simulink model "TestModel_2024a"  (R2024a)
settings: Solver=FixedStepAuto  StartTime=0.0  StopTime=4  FixedStep=1e-6  RelTol=1e-3
values from neighbouring files (symbols this model uses):
  pmsm = mcb.getPMSMParameters('Teknic2310P')    [mcb_pmsm_foc_sensorless_f28379d_datascript.m]
  Ts = T_pwm    (= 5e-05)    [mcb_pmsm_foc_sensorless_f28379d_datascript.m]
  Ts_motor = T_pwm/2    (= 2.5e-05)    [mcb_pmsm_foc_sensorless_f28379d_datascript.m]
undefined symbols (not defined in the file or in its folder): DiscIntNeverNeededParam
libraries: mcbcontrolslib x3, spsCurrentMeasurementLib x1, autolibim x1, spsPWMGenerator2LevelLib x1, eePwmGeneratorTwoLevel x1, spsThreePhaseVIMeasurementLib x1, spsTwoLevelConverterLib x1, spsDCVoltageSourceLib x1, spsVoltageMeasurementLib x1, spspowerguiLib x1
settings Model: Creator=ckb527612  LastModifiedBy=ckb527612
settings ConfigComp: CovBoundaryAbsTol=1.0e-5

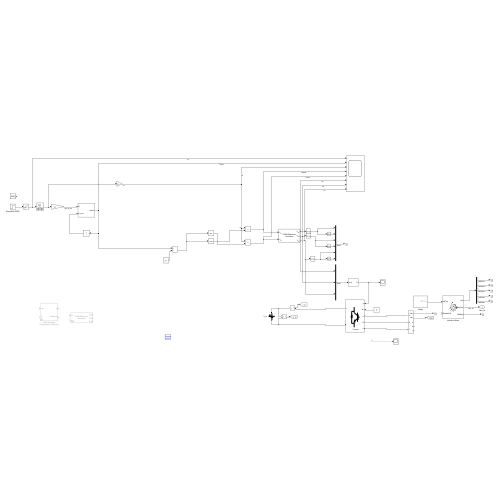
[thumbnail: Simulink's stored preview of the top-level diagram]
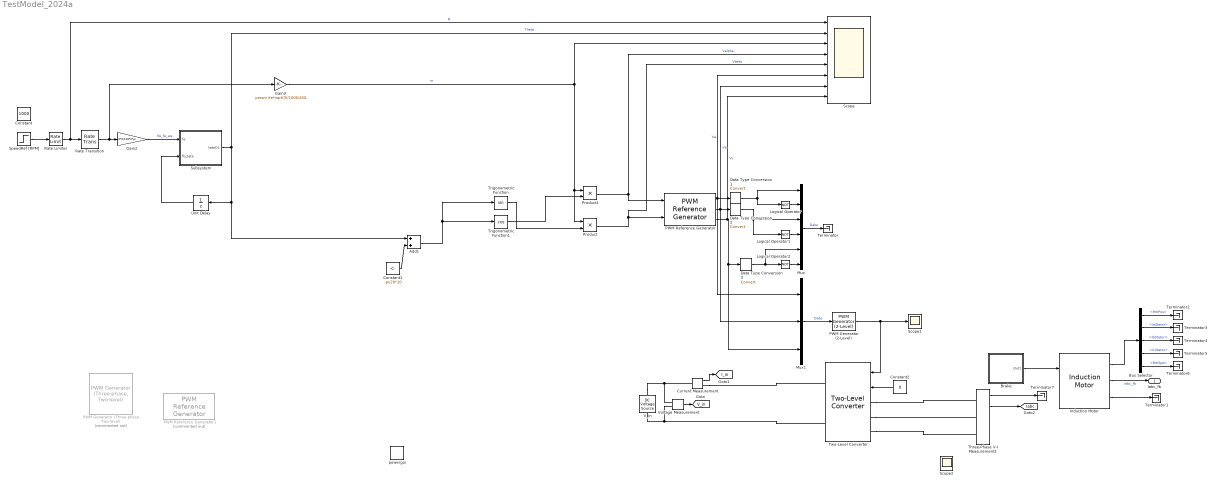
== system TestModel_2024a ==
  Add1 : Sum
  Brake : Subsystem
      mask Display: image('brake-system-types-and-hydraulic-brake-parts-and-functions-6.png');
  Bus Selector : BusSelector  OutputSignals=MtrPos,IaStator,IbStator,IcStator,MtrSpd
  Constant : Constant  Value=1000
  Constant1 : Constant  Value=-pi/20*10
  Constant2 : Constant  Value=0
  Current Measurement : spsCurrentMeasurementLib/Current Measurement  PhasorSimulation=off  OutputType=Complex  PSBequivalent=0
  Data Type Conversion1 : DataTypeConversion  SaturateOnIntegerOverflow=off  RndMeth=Floor
  Data Type Conversion2 : DataTypeConversion  SaturateOnIntegerOverflow=off  RndMeth=Floor
  Data Type Conversion3 : DataTypeConversion  SaturateOnIntegerOverflow=off  RndMeth=Floor
  Gain2 : Gain  Gain=2*2/120*2*pi
  Gain3 : Gain  Gain=pmsm.Ke*sqrt(3)/1000/450
  Induction Motor : autolibim/Induction Motor  sim_type=Discrete  Ts=0.001  port_config=Torque  P=2  Zs=[0.85 0.0139]  Zr="[0.55  0.0121]"  Lm=0.048  mechanical=[0.055 0.0078 0.5]  theta_init=0  omega_init=0  RefBlkName='autolibim/Induction Motor'  aMode=5
      settings: LibrarySourceBlock=mcblib/Electrical Systems/Motors/Induction Motor
  Logical Operator : Logic  Operator=NOT  AllPortsSameDT=off  OutDataTypeStr=boolean
  Logical Operator1 : Logic  Operator=NOT  AllPortsSameDT=off  OutDataTypeStr=boolean
  Logical Operator2 : Logic  Operator=NOT  AllPortsSameDT=off  OutDataTypeStr=boolean
  Mux : Mux  Inputs=6
  Mux1 : Mux  Inputs=3
  PWM Generator (2-Level) : spsPWMGenerator2LevelLib/PWM Generator (2-Level)  ModulatorType=Three-phase bridge (6 pulses)  ModulatorMode=Unsynchronized  Fc=10000  Pc=90  nF=27  MinMax="[ -1  1 ]"  SamplingTechnique=Natural  ModulatingSignals=off  m=0.8  Freq=60  Phase=0  Ts=1e-6  ShowCarrierOutport=off
  "PWM Generator (Three-phase, Two-level)" : eePwmGeneratorTwoLevel/PWM Generator (Three-phase, Two-level)  Commented=on  PWMMode=Continuous PWM (CPWM)  CPWMMode=SVM: space vector modulation  DPWMMode=60 DPWM: 60 degree discontinuous PWM  fsw=10e3  Ts=1e-6
      settings: LibrarySourceBlock=|
      | ee_sl_lib/Pulse Width
      | Modulation/PWM Generator
      | (Three-phase, Two-level)
  PWM Reference Generator : mcbcontrolslib/PWM Reference Generator  inSignal=Valphabeta  modType=SVM: space vector modulation
      settings: LibrarySourceBlock=mcblib/Controls/Math Transforms/PWM Reference Generator
  PWM Reference Generator1 : mcbcontrolslib/PWM Reference Generator  Commented=on  inSignal=Valphabeta  modType=SVM: space vector modulation
      settings: LibrarySourceBlock=mcblib/Controls/Math Transforms/PWM Reference Generator
  Product : Product
  Product1 : Product
  Rate Limiter : RateLimiter  RisingSlewLimit=1000  SampleTimeMode=inherited
  Rate Transition : RateTransition  OutPortSampleTime=5e-5
  Scope : Scope  NumInputPorts=8
  Scope1 : Scope
  Scope2 : Scope
  SpeedRef [RPM] : Step  Time=2  Before=500  After=1000  OutDataTypeStr=single  SampleTime=Ts
  Subsystem : Subsystem
  Terminator{,1..7} (8 alike) : Terminator
  Three-Phase V-I Measurement2 : spsThreePhaseVIMeasurementLib/Three-Phase V-I Measurement  VoltageMeasurement=phase-to-phase  SetLabelV=off  LabelV=Vabc  Vpu=off  VpuLL=off  CurrentMeasurement=yes  SetLabelI=off  LabelI=Iabc  Ipu=off  Pbase=100e6  Vbase=500e3  OutputType=Complex  PhasorSimulation=off  PSBequivalent=0
  Trigonometric Function : Trigonometry
  Trigonometric Function1 : Trigonometry  Operator=cos
  Two-Level Converter : spsTwoLevelConverterLib/Two-Level Converter  ModelType=Switching devices  Ron=1e-3  Rs=1e6  Cs=inf  Vforward=[0,0]  Ron_Diode=1e-3  Rs_Diode=1e6  Cs_Diode=inf  Vf_Diode=1e-3  Rs_CurrentSource=inf  Ron_ACsource=1e-3
      settings: LibrarySourceBlock=sps_lib/Power Electronics/Two-Level Converter
  Unit Delay : UnitDelay  SampleTime=-1  HasFrameUpgradeWarning=on
  "V_in " : spsDCVoltageSourceLib/DC Voltage Source  Amplitude=650  Measurements=None
  Voltage Measurement : spsVoltageMeasurementLib/Voltage Measurement  PhasorSimulation=off  OutputType=Complex  PSBequivalent=0
  powergui : spspowerguiLib/powergui  Priority=1  SimulationMode=Discrete  SampleTime=1e-6  frequency=60  Iterations=50  frequencyindice=0  Pbase=100e6  ErrMax=1e-4  UnitsV=kV  UnitsW=MW  buscounter=0  FunctionMessages=off  echomessages=off  EnableUseOfTLC=off  CurrentSourceSwitches=off  DisableSnubberDevices=off  DisableRonSwitches=off  DisableVfSwitches=off  DisplayEquations=off  AutomaticDiscreteSolvers=off  SolverType=Tustin/Backward Euler (TBE)  Interpol=off  ExternalGateDelay=off  methode=off  Ts=100  x0status=blocks  SPID=on  SwTol=0  HookPort=off  NonlinearTolerance=1e-4  nMaxIteration=100  ContinueOnMaxIteration=off  RestoreLinks=warning  ResistiveCurrentMeasurement=off  Frange=[0:2:500]  Ylog=off  Xlog=on  ShowGrid=off  save=off  variable=ZData  structure=0  ZoomFFT=off  StartTime=0.0  cycles=1  DisplayStyle=1  fundamental=60  FreqAxis=off  MaxFrequency=1000  frequencyindicesteady=1  RmsSteady=1  display=off
  Iabc_fb : Outport
  tag scope: I_in=global, Iabc=global, V_in=global
  wires:
  Unit Delay/1 -> Subsystem/2(fb_teta)
  Gain2/1 -> Subsystem/1(fe)  "Ns_fe_we"
  Rate Limiter/1 -> Scope/1, Rate Transition/1  "N"
  SpeedRef [RPM]/1 -> Rate Limiter/1
  Trigonometric Function1/1 -> Product1/2
  Data Type Conversion1/1 -> Logical Operator/1, Mux/1
  PWM Reference Generator/1 -> Mux1/1, Scope/6, Data Type Conversion1/1  "Va"
  Logical Operator1/1 -> Mux/4
  Data Type Conversion2/1 -> Logical Operator1/1, Mux/3
  Logical Operator2/1 -> Mux/6
  Product1/1 -> Scope/4, PWM Reference Generator/1  "Valpha"
  PWM Reference Generator/3 -> Scope/8, Mux1/3, Data Type Conversion3/1  "Vc"
  Trigonometric Function/1 -> Product/2
  PWM Reference Generator/2 -> Mux1/2, Scope/7, Data Type Conversion2/1  "Vb"
  Add1/1 -> Trigonometric Function1/1, Trigonometric Function/1
  Subsystem/1(tetaOL) -> Add1/1, Unit Delay/1, Scope/2  "Theta"
  Logical Operator/1 -> Mux/2
  Mux/1 -> Terminator/1  "Dabc"
  Product/1 -> Scope/5, PWM Reference Generator/2  "Vbeta"
  Data Type Conversion3/1 -> Mux/5, Logical Operator2/1
  Constant1/1 -> Add1/2
  Gain3/1 -> Product/1, Product1/1, Scope/3  "m"
  Rate Transition/1 -> Gain3/1, Gain2/1
  Mux1/1 -> PWM Generator (2-Level)/1  "Dabc"
  PWM Generator (2-Level)/1 -> Two-Level Converter/1, Scope1/1
  Constant2/1 -> Two-Level Converter/2
  Voltage Measurement/1 -> [V_in]
  Current Measurement/1 -> [I_in]
  Induction Motor/2 -> Iabc_fb/1  "Iabc_fb"
  Induction Motor/1 -> Bus Selector/1
  Three-Phase V-I Measurement2/1 -> Terminator7/1
  Three-Phase V-I Measurement2/2 -> [Iabc]
  Induction Motor/3 -> Terminator1/1
  Brake/1(Out1) -> Induction Motor/1
  Bus Selector/1 -> Terminator2/1  "<MtrPos>"
  Bus Selector/2 -> Terminator3/1  "<IaStator>"
  Bus Selector/3 -> Terminator4/1  "<IbStator>"
  Bus Selector/4 -> Terminator5/1  "<IcStator>"
  Bus Selector/5 -> Terminator6/1  "<MtrSpd>"
  ? -> Scope2/1
  connections:
  Voltage Measurement/LConn2 -- "V_in "/LConn1 -- Two-Level Converter/RConn2
  "V_in "/RConn1 -- Voltage Measurement/LConn1 -- Current Measurement/LConn1
  Current Measurement/RConn1 -- Two-Level Converter/RConn1
  Two-Level Converter/LConn1 -- Three-Phase V-I Measurement2/LConn1
  Two-Level Converter/LConn2 -- Three-Phase V-I Measurement2/LConn2
  Two-Level Converter/LConn3 -- Three-Phase V-I Measurement2/LConn3

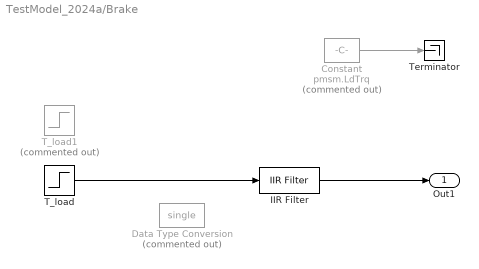
== system TestModel_2024a/Brake ==
  Constant : Constant  Commented=on  Value=pmsm.LdTrq
  Data Type Conversion : DataTypeConversion  Commented=on  OutDataTypeStr=single  SaturateOnIntegerOverflow=off  RndMeth=Floor
  IIR Filter : mcbcontrolslib/IIR Filter  VariantControl=Low Pass Filter  VariantSelect=Low-pass  FilterConstantInputType=Specify via dialog  Filter_constant=0.001  InitialOutput=Specify via dialog  InitialOutputValue=0  ExternalReset=none  advancedSettings=off  Ts=50e-6  cutOff_freq=3.1863
  T_load : Step  Time=2.5  Before=pmsm.T_rated*0  After=pmsm.T_rated*0.1  SampleTime=Ts_motor
  T_load1 : Step  Commented=on  Time=2.5  Before=pmsm.T_rated*0.1  After=pmsm.T_rated*0.5  SampleTime=Ts_motor
  Terminator : Terminator
  Out1 : Outport
  wires:
  Constant/1 -> Terminator/1
  T_load/1 -> IIR Filter/1
  IIR Filter/1 -> Out1/1

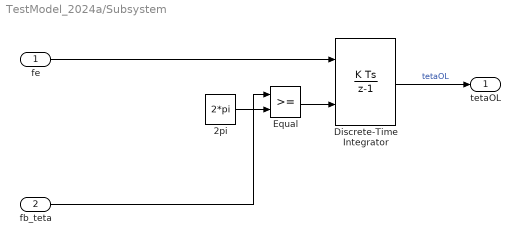
== system TestModel_2024a/Subsystem ==
  fe : Inport
  fb_teta : Inport  Port=2
  2pi : Constant  Value=2*pi
  Discrete-Time Integrator : DiscreteIntegrator  ExternalReset=rising  SampleTime=-1  LimitOutput=on  UpperSaturationLimit=2*pi  LowerSaturationLimit=0  ICPrevOutput=DiscIntNeverNeededParam  ICPrevScaledInput=DiscIntNeverNeededParam
  Equal : RelationalOperator  OutDataTypeStr=boolean  RndMeth=Simplest  InputSameDT=off
  tetaOL : Outport
  wires:
  fb_teta/1 -> Equal/1
  Equal/1 -> Discrete-Time Integrator/2
  2pi/1 -> Equal/2
  Discrete-Time Integrator/1 -> tetaOL/1  "tetaOL"
  fe/1 -> Discrete-Time Integrator/1
